simulink subsystem "Vorsteuerung_Fa_avRegler"  (R2020a)
settings: Solver=VariableStepAuto  StartTime=0.0  StopTime=10.0  RelTol=1e-3
model mask{K_p_v=0, a_max=0, regler=regler}
  mask prompts: K_p_v "a/v-Regler Kpv"; a_max "Soll-Beschleunigung Max (AW)"
undefined symbols (not defined in the file): kpv
settings Model: Creator=Tobias  LastModifiedBy=Tobias

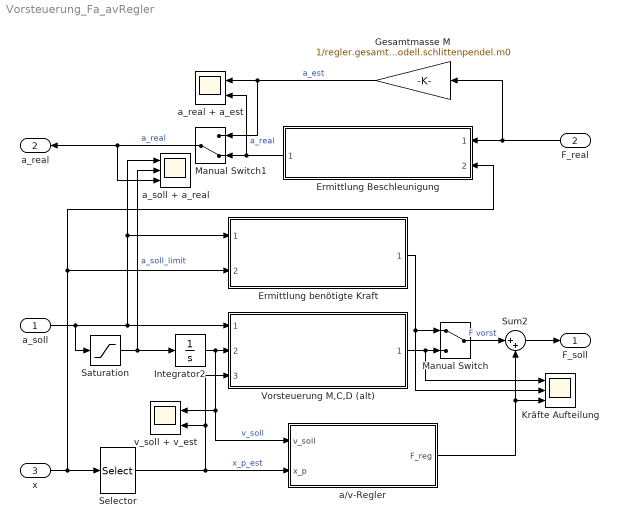
== system Vorsteuerung_Fa_avRegler ==
  a_soll : Inport
  F_real : Inport  Port=2
  x : Inport  Port=3
  Ermittlung Beschleunigung : Subsystem  ReferencedSubsystem=SchlittenGleichungBeschleunigung
  Ermittlung benötigte Kraft : Subsystem  ReferencedSubsystem=SchlittenGleichungKraft
  Gesamtmasse M : Gain  Gain=1/regler.gesamtmodell.schlittenpendel.m0
  Integrator2 : Integrator
  Kräfte Aufteilung : Scope  NumInputPorts=3
  Manual Switch : ManualSwitch
  Manual Switch1 : ManualSwitch  CurrentSetting=0
  Saturation : Saturate  UpperLimit=a_max  LowerLimit=-a_max
  Selector : Selector  InputPortWidth=6  IndexOptions=Index vector (dialog)  Indices=[2]  OutputSizes=1
  Sum2 : Sum  Inputs=|++
  Vorsteuerung M,C,D (alt) : Subsystem  ReferencedSubsystem=SchlittenVorsteuerung  SP=regler.gesamtmodell.schlittenpendel  vorst=regler.vorst
  a/v-Regler : Subsystem
  a_real + a_est : Scope  NumInputPorts=2
  a_soll + a_real : Scope  NumInputPorts=3
  v_soll + v_est : Scope  NumInputPorts=2
  F_soll : Outport
  a_real : Outport  Port=2
  wires:
  Selector/1 -> v_soll + v_est/2, Vorsteuerung M,C,D (alt)/3, a/v-Regler/2(x_p)  "x_p_est"
  Integrator2/1 -> v_soll + v_est/1, a/v-Regler/1(v_soll), Vorsteuerung M,C,D (alt)/2  "v_soll"
  a_soll/1 -> Saturation/1, a_soll + a_real/1, Ermittlung benötigte Kraft/1, Vorsteuerung M,C,D (alt)/1
  Sum2/1 -> F_soll/1
  Manual Switch/1 -> Sum2/1  "F vorst"
  x/1 -> Ermittlung Beschleunigung/2, Ermittlung benötigte Kraft/2, Selector/1
  a/v-Regler/1(F_reg) -> Kräfte Aufteilung/3, Sum2/2
  F_real/1 -> Gesamtmasse M/1, Ermittlung Beschleunigung/1
  Ermittlung Beschleunigung/1 -> a_real + a_est/2, Manual Switch1/2  "a_real"
  Ermittlung benötigte Kraft/1 -> Kräfte Aufteilung/2, Manual Switch/1
  Vorsteuerung M,C,D (alt)/1 -> Manual Switch/2, Kräfte Aufteilung/1
  Saturation/1 -> Integrator2/1, a_soll + a_real/2  "a_soll_limit"
  Gesamtmasse M/1 -> a_real + a_est/1, Manual Switch1/1  "a_est"
  Manual Switch1/1 -> a_real/1, a_soll + a_real/3  "a_real"

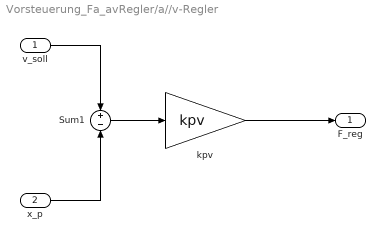
== system Vorsteuerung_Fa_avRegler/a//v-Regler ==
  v_soll : Inport
  x_p : Inport  Port=2
  Sum1 : Sum  Inputs=+|-
  kpv : Gain  Gain=kpv
  F_reg : Outport
  wires:
  Sum1/1 -> kpv/1
  x_p/1 -> Sum1/2
  v_soll/1 -> Sum1/1
  kpv/1 -> F_reg/1
